simulink model "day4"  (R2024a)
settings: Solver=VariableStepAuto  StartTime=0.0  StopTime=10.0  RelTol=1e-3
libraries: simulink_extras x17
settings Model: Creator=tusha  LastModifiedBy=tusha

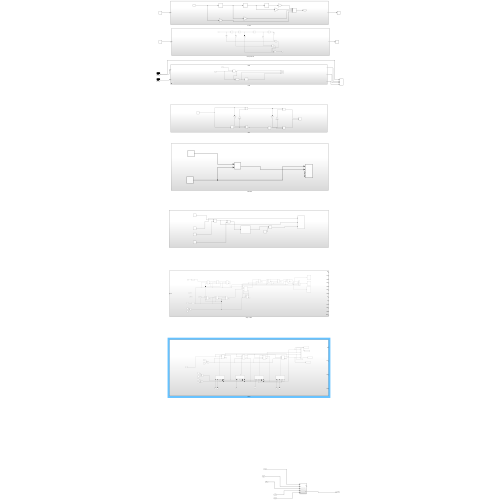
[thumbnail: Simulink's stored preview of the top-level diagram]
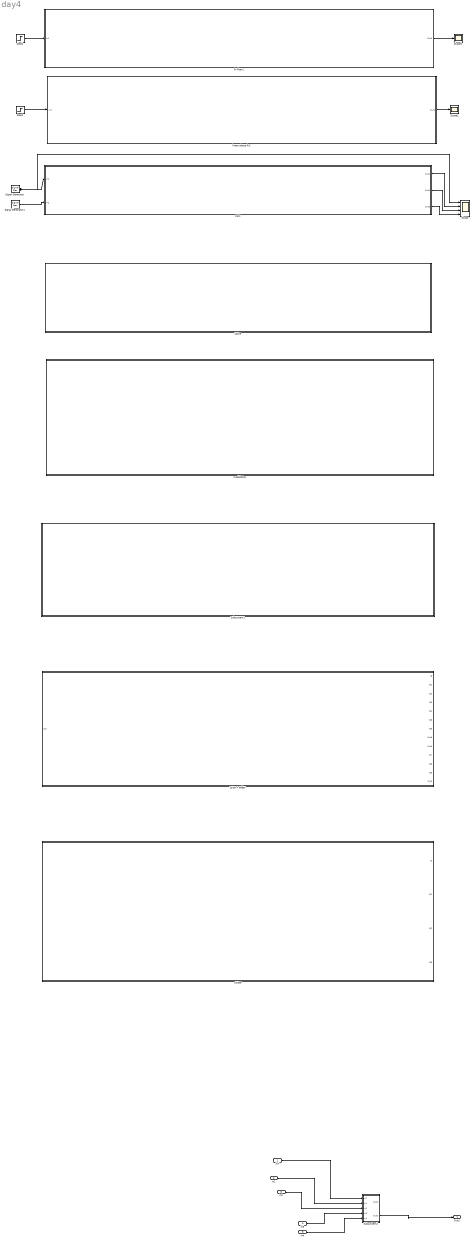
== system day4 ==
  In7 : Inport
  In1 : Inport  Port=2
  In2 : Inport  Port=3
  In3 : Inport  Port=4
  In4 : Inport  Port=5
  2sipo + adder : Subsystem
  PAM : Subsystem  Variant=on  VariantControlMode=label  VariantControl=PAM  LabelModeActiveChoice=PAM
  Scope : Scope  NumInputPorts=4
  Scope1 : Scope
  Scope2 : Scope
  Signal Generator : SignalGenerator  Units=rad/sec
  Signal Generator1 : SignalGenerator  WaveForm=square  Frequency=20  Units=rad/sec
  Step1 : Step  SampleTime=0
  Step2 : Step  SampleTime=0
  Subsystem1 : Subsystem
  Subsystem2 : Subsystem
  fir filter1 : Subsystem
  latice : Subsystem
  linear phase fir2 : Subsystem
  modulation : Subsystem
  shifter : Subsystem
  Out2 : Outport
  wires:
  Step1/1 -> fir filter1/1(In1)
  fir filter1/1(Out1) -> Scope1/1
  Step2/1 -> linear phase fir2/1(In1)
  linear phase fir2/1(Out1) -> Scope2/1
  Signal Generator/1 -> Scope/1, PAM/1(In1)
  Signal Generator1/1 -> PAM/2(In2)
  PAM/1(Out1) -> Scope/2
  PAM/2(Out2) -> Scope/3
  PAM/3(Out3) -> Scope/4
  In3/1 -> Subsystem2/4(In3)
  Subsystem2/2(Out2) -> Out2/1
  In1/1 -> Subsystem2/2(In1)
  In7/1 -> Subsystem2/1(In7)
  In2/1 -> Subsystem2/3(In2)
  In4/1 -> Subsystem2/5(In4)

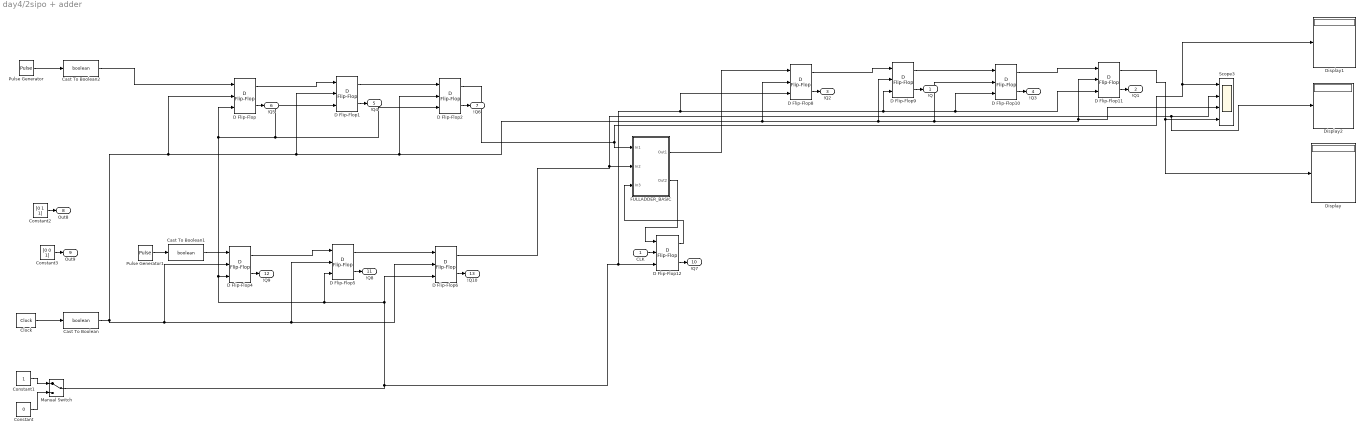
== system day4/2sipo + adder ==
  CLK : Inport
  Cast To Boolean : DataTypeConversion  OutDataTypeStr=boolean  SaturateOnIntegerOverflow=off  RndMeth=Floor
  Cast To Boolean1 : DataTypeConversion  OutDataTypeStr=boolean  SaturateOnIntegerOverflow=off  RndMeth=Floor
  Cast To Boolean2 : DataTypeConversion  OutDataTypeStr=boolean  SaturateOnIntegerOverflow=off  RndMeth=Floor
  Clock : simulink_extras/Flip Flops/Clock  period=0.5
  Constant : Constant  Value=0  OutDataTypeStr=boolean
  Constant1 : Constant  OutDataTypeStr=boolean
  Constant2 : Constant  Value=[0 1 1]
  Constant3 : Constant  Value=[0 0 1]
  D Flip-Flop{,1..2,4..6,8..12} (11 alike) : simulink_extras/Flip Flops/D Flip-Flop
  Display : Display
  Display1 : Display
  Display2 : Display
  FULLADDER_BASIC : Subsystem
  Manual Switch : ManualSwitch
  Pulse Generator : DiscretePulseGenerator  PulseType=Time based  PulseWidth=50
  Pulse Generator1 : DiscretePulseGenerator  PulseType=Time based  Period=1  PulseWidth=50
  Scope3 : Scope  NumInputPorts=4
  !Q : Outport
  !Q1 : Outport  Port=2
  !Q2 : Outport  Port=3
  !Q3 : Outport  Port=4
  !Q4 : Outport  Port=5
  !Q5 : Outport  Port=6
  !Q6 : Outport  Port=7
  Out8 : Outport  Port=8
  Out9 : Outport  Port=9
  !Q7 : Outport  Port=10
  !Q8 : Outport  Port=11
  !Q9 : Outport  Port=12
  !Q10 : Outport  Port=13
  wires:
  Cast To Boolean/1 -> D Flip-Flop6/2, D Flip-Flop5/2, D Flip-Flop4/2, Scope3/3, D Flip-Flop11/2, D Flip-Flop10/2, D Flip-Flop9/2, D Flip-Flop8/2, D Flip-Flop2/2, D Flip-Flop1/2, D Flip-Flop/2
  D Flip-Flop10/1 -> D Flip-Flop11/1
  Manual Switch/1 -> D Flip-Flop8/3, D Flip-Flop9/3, D Flip-Flop10/3, D Flip-Flop11/3, D Flip-Flop12/3, D Flip-Flop6/3, D Flip-Flop2/3, D Flip-Flop1/3, D Flip-Flop/3, D Flip-Flop4/3, D Flip-Flop5/3
  D Flip-Flop8/1 -> D Flip-Flop9/1
  D Flip-Flop11/1 -> Scope3/4, Display/1
  Pulse Generator/1 -> Cast To Boolean2/1
  Clock/1 -> Cast To Boolean/1
  D Flip-Flop4/1 -> D Flip-Flop5/1
  Constant2/1 -> Out8/1
  Cast To Boolean2/1 -> D Flip-Flop/1
  D Flip-Flop9/1 -> D Flip-Flop10/1
  D Flip-Flop5/1 -> D Flip-Flop6/1
  D Flip-Flop1/1 -> D Flip-Flop2/1
  D Flip-Flop6/1 -> FULLADDER_BASIC/2(In2), Scope3/2, Display2/1
  D Flip-Flop2/1 -> FULLADDER_BASIC/1(In1), Scope3/1, Display1/1
  D Flip-Flop/1 -> D Flip-Flop1/1
  Constant/1 -> Manual Switch/2
  D Flip-Flop8/2 -> !Q2/1
  D Flip-Flop12/1 -> FULLADDER_BASIC/3(In3)
  Pulse Generator1/1 -> Cast To Boolean1/1
  FULLADDER_BASIC/2(Out2) -> D Flip-Flop12/1
  FULLADDER_BASIC/1(Out1) -> D Flip-Flop8/1
  Constant1/1 -> Manual Switch/1
  Cast To Boolean1/1 -> D Flip-Flop4/1
  D Flip-Flop10/2 -> !Q3/1
  D Flip-Flop11/2 -> !Q1/1
  D Flip-Flop4/2 -> !Q9/1
  D Flip-Flop9/2 -> !Q/1
  D Flip-Flop5/2 -> !Q8/1
  D Flip-Flop1/2 -> !Q4/1
  CLK/1 -> D Flip-Flop12/2
  D Flip-Flop6/2 -> !Q10/1
  D Flip-Flop12/2 -> !Q7/1
  D Flip-Flop/2 -> !Q5/1
  D Flip-Flop2/2 -> !Q6/1
  Constant3/1 -> Out9/1

== system day4/PAM ==
  In1 : Inport
  In2 : Inport  Port=2
  PAM : Subsystem  VariantControl=PAM
  Out1 : Outport
  Out2 : Outport  Port=2
  Out3 : Outport  Port=3

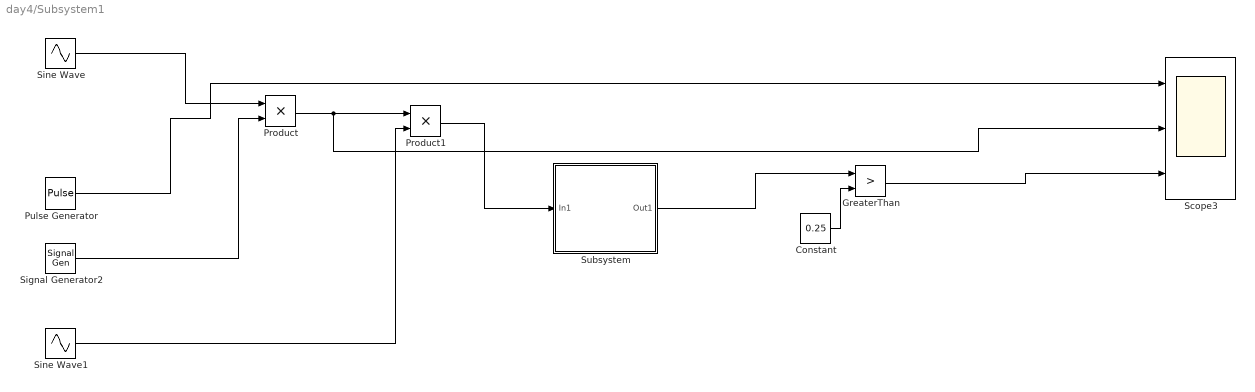
== system day4/Subsystem1 ==
  Constant : Constant  Value=0.25
  GreaterThan : RelationalOperator  Operator=>  OutDataTypeStr=boolean  RndMeth=Simplest  InputSameDT=off
  Product : Product
  Product1 : Product
  Pulse Generator : DiscretePulseGenerator  PulseType=Time based  Period=1  PulseWidth=50
  Scope3 : Scope  NumInputPorts=3
  Signal Generator2 : SignalGenerator  Units=rad/sec
  Sine Wave : Sin  Frequency=20  SampleTime=0
  Sine Wave1 : Sin  Frequency=20  SampleTime=0
  Subsystem : Subsystem
  wires:
  Pulse Generator/1 -> Scope3/1
  Sine Wave1/1 -> Product1/2
  Signal Generator2/1 -> Product/2
  Sine Wave/1 -> Product/1
  Subsystem/1(Out1) -> GreaterThan/1
  Product1/1 -> Subsystem/1(In1)
  Constant/1 -> GreaterThan/2
  Product/1 -> Scope3/2, Product1/1
  GreaterThan/1 -> Scope3/3

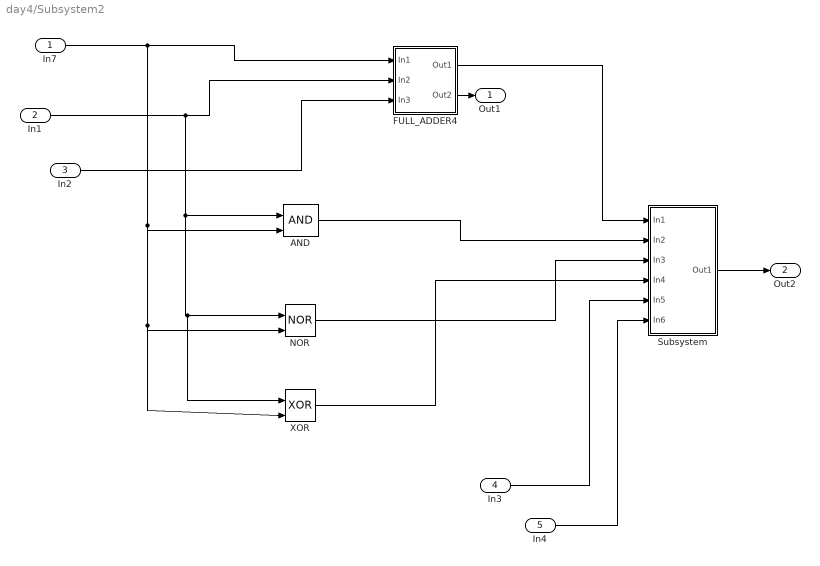
== system day4/Subsystem2 ==
  In7 : Inport
  In1 : Inport  Port=2
  In2 : Inport  Port=3
  In3 : Inport  Port=4
  In4 : Inport  Port=5
  AND : Logic  IconShape=distinctive  AllPortsSameDT=off  OutDataTypeStr=boolean
  FULL_ADDER4 : Subsystem
  NOR : Logic  Operator=NOR  IconShape=distinctive  AllPortsSameDT=off  OutDataTypeStr=boolean
  Subsystem : Subsystem
  XOR : Logic  Operator=XOR  IconShape=distinctive  AllPortsSameDT=off  OutDataTypeStr=boolean
  Out1 : Outport
  Out2 : Outport  Port=2
  wires:
  In7/1 -> XOR/2, NOR/2, AND/2, FULL_ADDER4/1(In1)
  Subsystem/1(Out1) -> Out2/1
  FULL_ADDER4/1(Out1) -> Subsystem/1(In1)
  In4/1 -> Subsystem/6(In6)
  In1/1 -> XOR/1, NOR/1, AND/1, FULL_ADDER4/2(In2)
  In2/1 -> FULL_ADDER4/3(In3)
  XOR/1 -> Subsystem/4(In4)
  AND/1 -> Subsystem/2(In2)
  NOR/1 -> Subsystem/3(In3)
  In3/1 -> Subsystem/5(In5)
  FULL_ADDER4/2(Out2) -> Out1/1

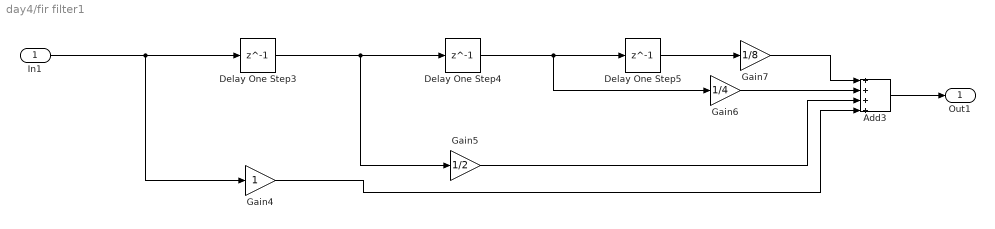
== system day4/fir filter1 ==
  In1 : Inport
  Add3 : Sum  Inputs=++++
  Delay One Step3 : Delay  DelayLength=1
  Delay One Step4 : Delay  DelayLength=1
  Delay One Step5 : Delay  DelayLength=1
  Gain4 : Gain
  Gain5 : Gain  Gain=1/2
  Gain6 : Gain  Gain=1/4
  Gain7 : Gain  Gain=1/8
  Out1 : Outport
  wires:
  Delay One Step5/1 -> Gain7/1
  Delay One Step4/1 -> Delay One Step5/1, Gain6/1
  Gain4/1 -> Add3/4
  Gain7/1 -> Add3/1
  Delay One Step3/1 -> Delay One Step4/1, Gain5/1
  Gain6/1 -> Add3/2
  Gain5/1 -> Add3/3
  In1/1 -> Gain4/1, Delay One Step3/1
  Add3/1 -> Out1/1

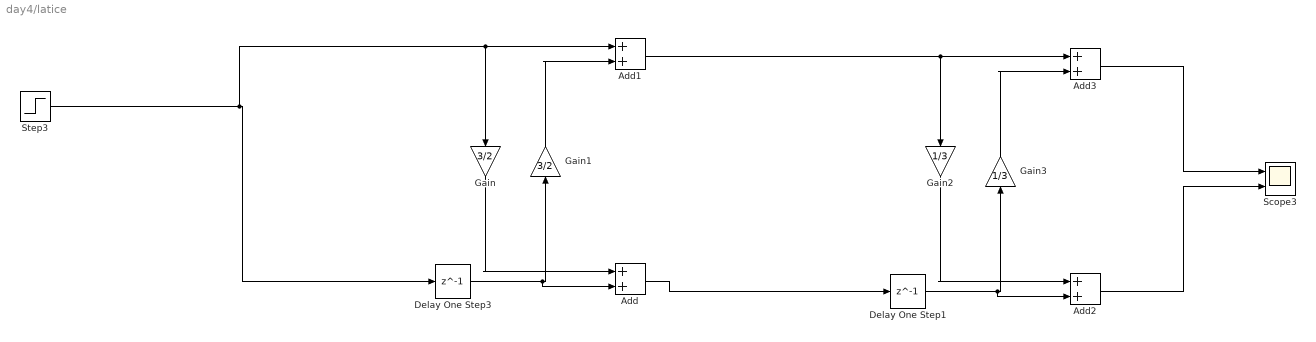
== system day4/latice ==
  Add{,1..3} (4 alike) : Sum
  Delay One Step1 : Delay  DelayLength=1
  Delay One Step3 : Delay  DelayLength=1
  Gain : Gain  Gain=3/2
  Gain1 : Gain  Gain=3/2
  Gain2 : Gain  Gain=1/3
  Gain3 : Gain  Gain=1/3
  Scope3 : Scope  NumInputPorts=2
  Step3 : Step  SampleTime=0
  wires:
  Add2/1 -> Scope3/2
  Gain1/1 -> Add1/2
  Gain3/1 -> Add3/2
  Step3/1 -> Gain/1, Add1/1, Delay One Step3/1
  Delay One Step3/1 -> Add/2, Gain1/1
  Gain/1 -> Add/1
  Add/1 -> Delay One Step1/1
  Delay One Step1/1 -> Add2/2, Gain3/1
  Add3/1 -> Scope3/1
  Gain2/1 -> Add2/1
  Add1/1 -> Gain2/1, Add3/1

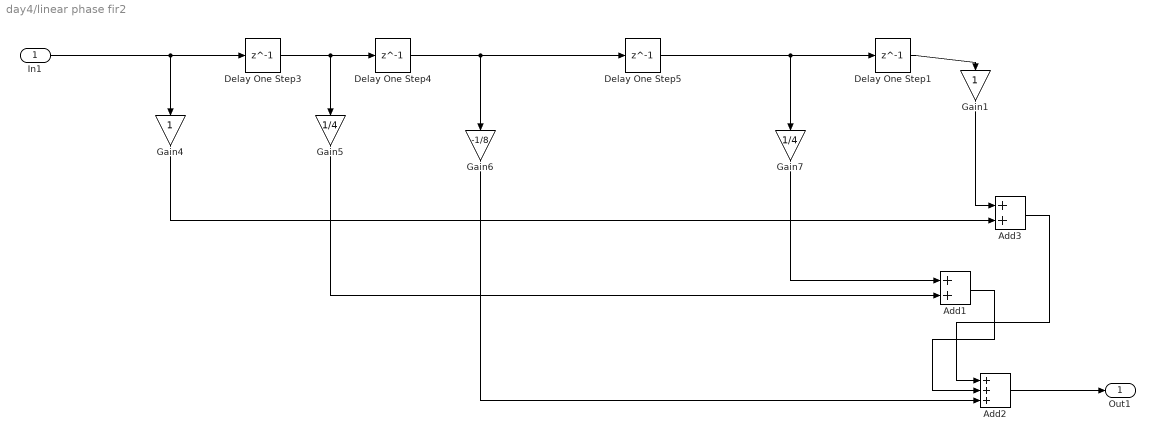
== system day4/linear phase fir2 ==
  In1 : Inport
  Add1 : Sum
  Add2 : Sum  Inputs=+++
  Add3 : Sum
  Delay One Step{1,3..5} (4 alike) : Delay  DelayLength=1
  Gain1 : Gain
  Gain4 : Gain
  Gain5 : Gain  Gain=1/4
  Gain6 : Gain  Gain=-1/8
  Gain7 : Gain  Gain=1/4
  Out1 : Outport
  wires:
  Delay One Step4/1 -> Delay One Step5/1, Gain6/1
  Add3/1 -> Add2/1
  Add1/1 -> Add2/2
  Delay One Step5/1 -> Delay One Step1/1, Gain7/1
  In1/1 -> Gain4/1, Delay One Step3/1
  Delay One Step3/1 -> Delay One Step4/1, Gain5/1
  Gain4/1 -> Add3/2
  Gain6/1 -> Add2/3
  Delay One Step1/1 -> Gain1/1
  Gain7/1 -> Add1/1
  Gain5/1 -> Add1/2
  Gain1/1 -> Add3/1
  Add2/1 -> Out1/1

== system day4/modulation ==
  Product : Product
  Pulse Generator : DiscretePulseGenerator  PulseType=Time based  Period=1  PulseWidth=50
  Scope3 : Scope  NumInputPorts=4
  Sine Wave : Sin  Frequency=50  SampleTime=0
  wires:
  Sine Wave/1 -> Product/1
  Pulse Generator/1 -> Scope3/1, Product/2
  Product/1 -> Scope3/2

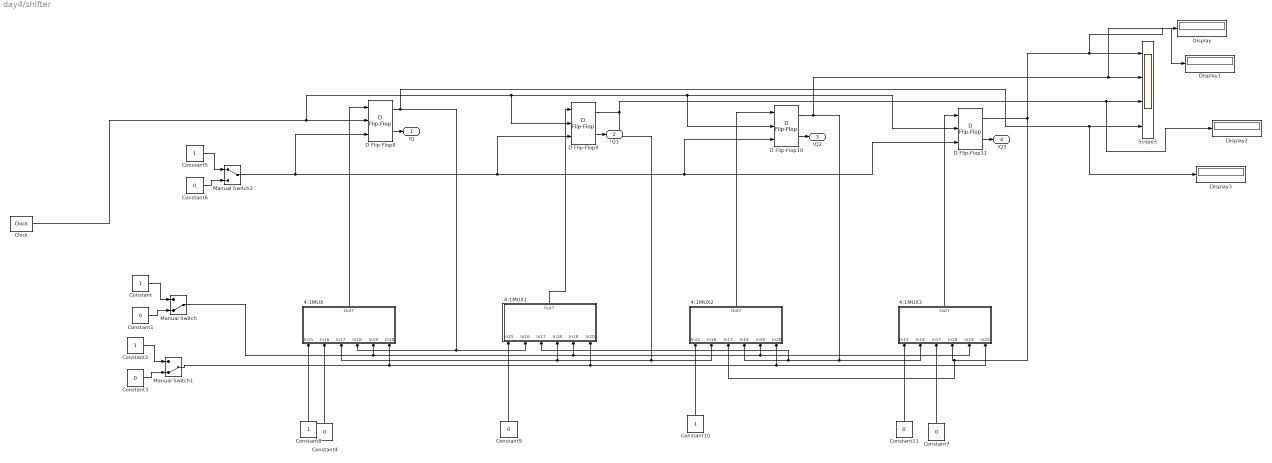
== system day4/shifter ==
  4:1MUX : Subsystem
  4:1MUX1 : Subsystem
  4:1MUX2 : Subsystem
  4:1MUX3 : Subsystem
  Clock : simulink_extras/Flip Flops/Clock  period=2
  Constant{,2,5,8,10} (5 alike) : Constant
  Constant{1,3..4,6..7,9,11} (7 alike) : Constant  Value=0
  D Flip-Flop{8..11} (4 alike) : simulink_extras/Flip Flops/D Flip-Flop
  Display{,1..3} (4 alike) : Display
  Manual Switch : ManualSwitch  CurrentSetting=0
  Manual Switch1 : ManualSwitch  CurrentSetting=0
  Manual Switch2 : ManualSwitch
  Scope3 : Scope  NumInputPorts=4
  !Q : Outport
  !Q1 : Outport  Port=2
  !Q2 : Outport  Port=3
  !Q3 : Outport  Port=4
  wires:
  4:1MUX2/1(Out7) -> D Flip-Flop10/1
  Constant/1 -> Manual Switch/1
  Constant8/1 -> 4:1MUX/1(In15)
  Manual Switch2/1 -> D Flip-Flop11/3, D Flip-Flop10/3, D Flip-Flop9/3, D Flip-Flop8/3
  Manual Switch/1 -> 4:1MUX3/5(In19), 4:1MUX2/5(In19), 4:1MUX1/5(In19), 4:1MUX/5(In19)
  4:1MUX3/1(Out7) -> D Flip-Flop11/1
  D Flip-Flop11/1 -> 4:1MUX2/3(In17), 4:1MUX3/4(In18), Display/1, Scope3/1
  D Flip-Flop9/1 -> 4:1MUX/3(In17), 4:1MUX1/4(In18), 4:1MUX2/2(In16), Display2/1, Scope3/3
  D Flip-Flop9/2 -> !Q1/1
  4:1MUX1/1(Out7) -> D Flip-Flop9/1
  Manual Switch1/1 -> 4:1MUX/6(In20), 4:1MUX1/6(In20), 4:1MUX3/6(In20), 4:1MUX2/6(In20)
  D Flip-Flop10/1 -> Display1/1, Scope3/2, 4:1MUX1/3(In17), 4:1MUX2/4(In18), 4:1MUX3/2(In16)
  Constant3/1 -> Manual Switch1/2
  D Flip-Flop8/1 -> Display3/1, Scope3/4, 4:1MUX1/2(In16), 4:1MUX/4(In18)
  Constant6/1 -> Manual Switch2/2
  Constant2/1 -> Manual Switch1/1
  Constant5/1 -> Manual Switch2/1
  Constant9/1 -> 4:1MUX1/1(In15)
  Clock/1 -> D Flip-Flop10/2, D Flip-Flop11/2, D Flip-Flop9/2, D Flip-Flop8/2
  Constant7/1 -> 4:1MUX3/3(In17)
  Constant4/1 -> 4:1MUX/2(In16)
  Constant1/1 -> Manual Switch/2
  4:1MUX/1(Out7) -> D Flip-Flop8/1
  Constant10/1 -> 4:1MUX2/1(In15)
  Constant11/1 -> 4:1MUX3/1(In15)
  D Flip-Flop10/2 -> !Q2/1
  D Flip-Flop11/2 -> !Q3/1
  D Flip-Flop8/2 -> !Q/1

== system day4/2sipo + adder/FULLADDER_BASIC ==
  In1 : Inport
  In2 : Inport  Port=2
  In3 : Inport  Port=3
  HA_Basic1 : Subsystem
  HA_Basic2 : Subsystem
  Logical Operator4 : Logic  Operator=OR  IconShape=distinctive  AllPortsSameDT=off  OutDataTypeStr=boolean
  Out1 : Outport
  Out2 : Outport  Port=2
  wires:
  HA_Basic1/1(Out1) -> HA_Basic2/1(In1)
  HA_Basic1/2(Out2) -> Logical Operator4/2
  HA_Basic2/2(Out2) -> Logical Operator4/1
  In1/1 -> HA_Basic1/1(In1)
  Logical Operator4/1 -> Out2/1
  In2/1 -> HA_Basic1/2(In2)
  HA_Basic2/1(Out1) -> Out1/1
  In3/1 -> HA_Basic2/2(In2)

== system day4/PAM/PAM ==
  In1 : Inport
  In2 : Inport  Port=2
  Product : Product
  Product1 : Product
  fir filter2 : Subsystem
  Out1 : Outport
  Out2 : Outport  Port=2
  Out3 : Outport  Port=3
  wires:
  fir filter2/1(Out1) -> Out3/1
  Product/1 -> Out1/1, Product1/1
  In2/1 -> Product/2, Product1/2
  In1/1 -> Product/1
  Product1/1 -> Out2/1, fir filter2/1(In1)

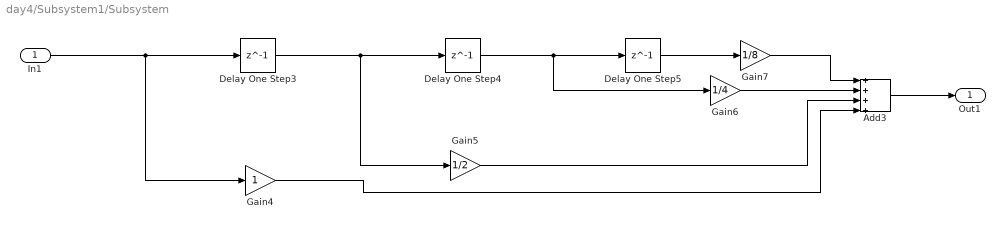
== system day4/Subsystem1/Subsystem ==
  In1 : Inport
  Add3 : Sum  Inputs=++++
  Delay One Step3 : Delay  DelayLength=1
  Delay One Step4 : Delay  DelayLength=1
  Delay One Step5 : Delay  DelayLength=1
  Gain4 : Gain
  Gain5 : Gain  Gain=1/2
  Gain6 : Gain  Gain=1/4
  Gain7 : Gain  Gain=1/8
  Out1 : Outport
  wires:
  Gain6/1 -> Add3/2
  In1/1 -> Gain4/1, Delay One Step3/1
  Delay One Step4/1 -> Delay One Step5/1, Gain6/1
  Gain4/1 -> Add3/4
  Gain5/1 -> Add3/3
  Delay One Step5/1 -> Gain7/1
  Delay One Step3/1 -> Delay One Step4/1, Gain5/1
  Gain7/1 -> Add3/1
  Add3/1 -> Out1/1

== system day4/Subsystem2/FULL_ADDER4 ==
  In1 : Inport
  In2 : Inport  Port=2
  In3 : Inport  Port=3
  Logical Operator : Logic  Operator=OR  AllPortsSameDT=off  OutDataTypeStr=boolean
  half_adder : Subsystem
  half_adder1 : Subsystem
  Out1 : Outport
  Out2 : Outport  Port=2
  wires:
  half_adder1/2(Out2) -> Logical Operator/2
  In3/1 -> half_adder1/2(In2)
  In1/1 -> half_adder/1(In1)
  half_adder1/1(Out1) -> Out1/1
  half_adder/1(Out1) -> half_adder1/1(In1)
  half_adder/2(Out2) -> Logical Operator/1
  In2/1 -> half_adder/2(In2)
  Logical Operator/1 -> Out2/1

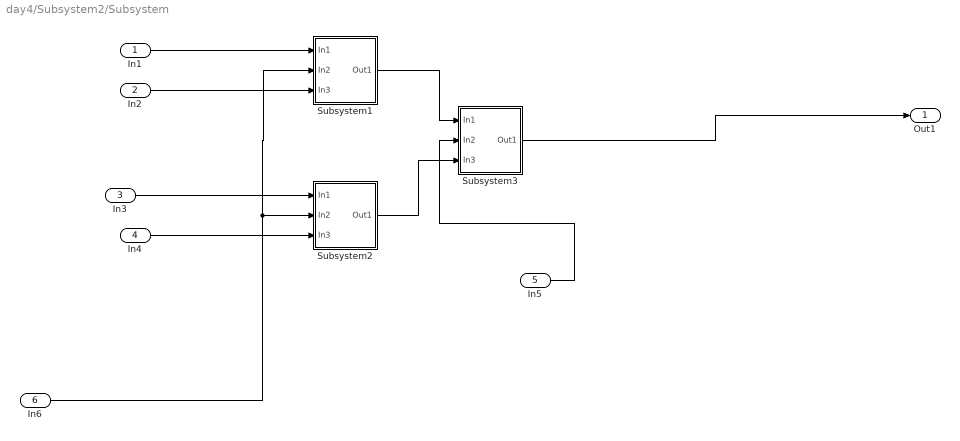
== system day4/Subsystem2/Subsystem ==
  In1 : Inport
  In2 : Inport  Port=2
  In3 : Inport  Port=3
  In4 : Inport  Port=4
  In5 : Inport  Port=5
  In6 : Inport  Port=6
  Subsystem1 : Subsystem
  Subsystem2 : Subsystem
  Subsystem3 : Subsystem
  Out1 : Outport
  wires:
  In6/1 -> Subsystem1/2(In2), Subsystem2/2(In2)
  In2/1 -> Subsystem1/3(In3)
  In3/1 -> Subsystem2/1(In1)
  Subsystem2/1(Out1) -> Subsystem3/3(In3)
  Subsystem1/1(Out1) -> Subsystem3/1(In1)
  In4/1 -> Subsystem2/3(In3)
  In1/1 -> Subsystem1/1(In1)
  In5/1 -> Subsystem3/2(In2)
  Subsystem3/1(Out1) -> Out1/1

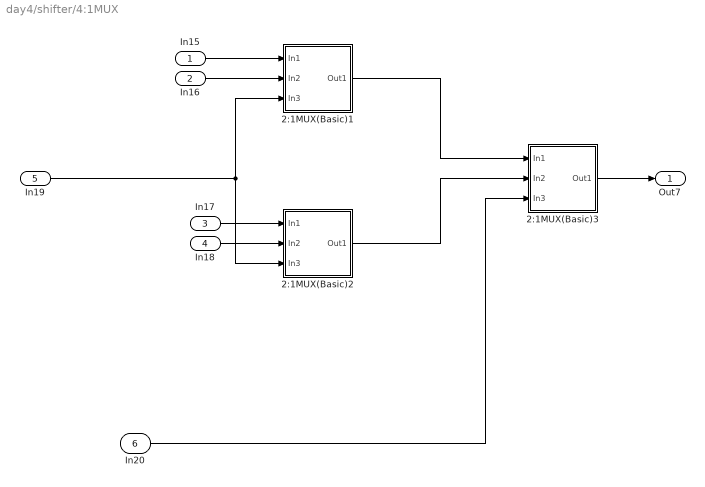
== system day4/shifter/4:1MUX ==
  In15 : Inport
  In16 : Inport  Port=2
  In17 : Inport  Port=3
  In18 : Inport  Port=4
  In19 : Inport  Port=5
  In20 : Inport  Port=6
  2:1MUX(Basic)1 : Subsystem
  2:1MUX(Basic)2 : Subsystem
  2:1MUX(Basic)3 : Subsystem
  Out7 : Outport
  wires:
  In18/1 -> 2:1MUX(Basic)2/2(In2)
  In16/1 -> 2:1MUX(Basic)1/2(In2)
  In17/1 -> 2:1MUX(Basic)2/1(In1)
  In19/1 -> 2:1MUX(Basic)2/3(In3), 2:1MUX(Basic)1/3(In3)
  2:1MUX(Basic)2/1(Out1) -> 2:1MUX(Basic)3/2(In2)
  2:1MUX(Basic)1/1(Out1) -> 2:1MUX(Basic)3/1(In1)
  In20/1 -> 2:1MUX(Basic)3/3(In3)
  In15/1 -> 2:1MUX(Basic)1/1(In1)
  2:1MUX(Basic)3/1(Out1) -> Out7/1

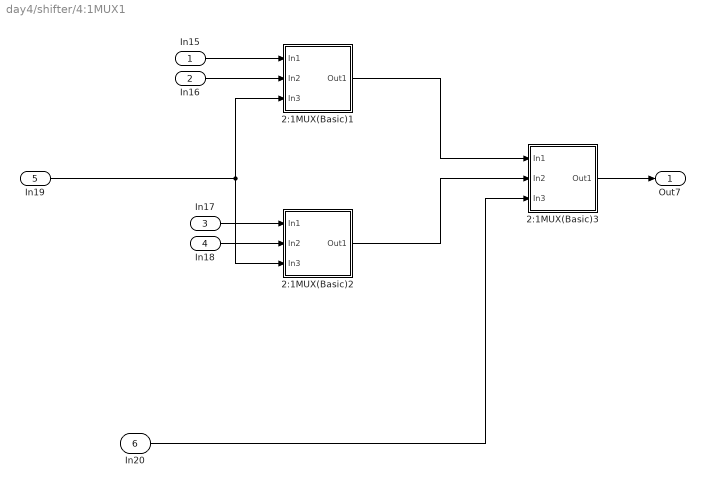
== system day4/shifter/4:1MUX1 ==
  In15 : Inport
  In16 : Inport  Port=2
  In17 : Inport  Port=3
  In18 : Inport  Port=4
  In19 : Inport  Port=5
  In20 : Inport  Port=6
  2:1MUX(Basic)1 : Subsystem
  2:1MUX(Basic)2 : Subsystem
  2:1MUX(Basic)3 : Subsystem
  Out7 : Outport
  wires:
  In18/1 -> 2:1MUX(Basic)2/2(In2)
  In16/1 -> 2:1MUX(Basic)1/2(In2)
  In17/1 -> 2:1MUX(Basic)2/1(In1)
  In19/1 -> 2:1MUX(Basic)2/3(In3), 2:1MUX(Basic)1/3(In3)
  2:1MUX(Basic)2/1(Out1) -> 2:1MUX(Basic)3/2(In2)
  2:1MUX(Basic)1/1(Out1) -> 2:1MUX(Basic)3/1(In1)
  In20/1 -> 2:1MUX(Basic)3/3(In3)
  In15/1 -> 2:1MUX(Basic)1/1(In1)
  2:1MUX(Basic)3/1(Out1) -> Out7/1

== system day4/shifter/4:1MUX2 ==
  In15 : Inport
  In16 : Inport  Port=2
  In17 : Inport  Port=3
  In18 : Inport  Port=4
  In19 : Inport  Port=5
  In20 : Inport  Port=6
  2:1MUX(Basic)1 : Subsystem
  2:1MUX(Basic)2 : Subsystem
  2:1MUX(Basic)3 : Subsystem
  Out7 : Outport
  wires:
  In18/1 -> 2:1MUX(Basic)2/2(In2)
  In16/1 -> 2:1MUX(Basic)1/2(In2)
  In17/1 -> 2:1MUX(Basic)2/1(In1)
  In19/1 -> 2:1MUX(Basic)2/3(In3), 2:1MUX(Basic)1/3(In3)
  2:1MUX(Basic)2/1(Out1) -> 2:1MUX(Basic)3/2(In2)
  2:1MUX(Basic)1/1(Out1) -> 2:1MUX(Basic)3/1(In1)
  In20/1 -> 2:1MUX(Basic)3/3(In3)
  In15/1 -> 2:1MUX(Basic)1/1(In1)
  2:1MUX(Basic)3/1(Out1) -> Out7/1

== system day4/shifter/4:1MUX3 ==
  In15 : Inport
  In16 : Inport  Port=2
  In17 : Inport  Port=3
  In18 : Inport  Port=4
  In19 : Inport  Port=5
  In20 : Inport  Port=6
  2:1MUX(Basic)1 : Subsystem
  2:1MUX(Basic)2 : Subsystem
  2:1MUX(Basic)3 : Subsystem
  Out7 : Outport
  wires:
  In18/1 -> 2:1MUX(Basic)2/2(In2)
  In16/1 -> 2:1MUX(Basic)1/2(In2)
  In17/1 -> 2:1MUX(Basic)2/1(In1)
  In19/1 -> 2:1MUX(Basic)2/3(In3), 2:1MUX(Basic)1/3(In3)
  2:1MUX(Basic)2/1(Out1) -> 2:1MUX(Basic)3/2(In2)
  2:1MUX(Basic)1/1(Out1) -> 2:1MUX(Basic)3/1(In1)
  In20/1 -> 2:1MUX(Basic)3/3(In3)
  In15/1 -> 2:1MUX(Basic)1/1(In1)
  2:1MUX(Basic)3/1(Out1) -> Out7/1

== system day4/2sipo + adder/FULLADDER_BASIC/HA_Basic1 ==
  In1 : Inport
  In2 : Inport  Port=2
  Logical Operator2 : Logic  IconShape=distinctive  AllPortsSameDT=off  OutDataTypeStr=boolean
  XOR_basic1 : Subsystem
  Out1 : Outport
  Out2 : Outport  Port=2
  wires:
  XOR_basic1/1(Out1) -> Out1/1
  Logical Operator2/1 -> Out2/1
  In1/1 -> Logical Operator2/1, XOR_basic1/1(In1)
  In2/1 -> Logical Operator2/2, XOR_basic1/2(In2)

== system day4/2sipo + adder/FULLADDER_BASIC/HA_Basic2 ==
  In1 : Inport
  In2 : Inport  Port=2
  Logical Operator2 : Logic  IconShape=distinctive  AllPortsSameDT=off  OutDataTypeStr=boolean
  XOR_basic1 : Subsystem
  Out1 : Outport
  Out2 : Outport  Port=2
  wires:
  XOR_basic1/1(Out1) -> Out1/1
  Logical Operator2/1 -> Out2/1
  In1/1 -> Logical Operator2/1, XOR_basic1/1(In1)
  In2/1 -> Logical Operator2/2, XOR_basic1/2(In2)

== system day4/PAM/PAM/fir filter2 ==
  In1 : Inport
  Add3 : Sum  Inputs=++++
  Delay One Step3 : Delay  DelayLength=1
  Delay One Step4 : Delay  DelayLength=1
  Delay One Step5 : Delay  DelayLength=1
  Gain4 : Gain
  Gain5 : Gain  Gain=1/2
  Gain6 : Gain  Gain=1/4
  Gain7 : Gain  Gain=1/8
  Out1 : Outport
  wires:
  Delay One Step5/1 -> Gain7/1
  Delay One Step4/1 -> Delay One Step5/1, Gain6/1
  Gain4/1 -> Add3/4
  Gain7/1 -> Add3/1
  Delay One Step3/1 -> Delay One Step4/1, Gain5/1
  Gain6/1 -> Add3/2
  Gain5/1 -> Add3/3
  In1/1 -> Gain4/1, Delay One Step3/1
  Add3/1 -> Out1/1

== system day4/Subsystem2/FULL_ADDER4/half_adder ==
  In1 : Inport
  In2 : Inport  Port=2
  Logical Operator1 : Logic  AllPortsSameDT=off  OutDataTypeStr=boolean
  XOR_BASIC : Subsystem
  Out1 : Outport
  Out2 : Outport  Port=2
  wires:
  In1/1 -> XOR_BASIC/1(In1), Logical Operator1/1
  In2/1 -> XOR_BASIC/2(In2), Logical Operator1/2
  Logical Operator1/1 -> Out2/1
  XOR_BASIC/1(Out1) -> Out1/1

== system day4/Subsystem2/FULL_ADDER4/half_adder1 ==
  In1 : Inport
  In2 : Inport  Port=2
  Logical Operator1 : Logic  AllPortsSameDT=off  OutDataTypeStr=boolean
  XOR_BASIC : Subsystem
  Out1 : Outport
  Out2 : Outport  Port=2
  wires:
  In1/1 -> XOR_BASIC/1(In1), Logical Operator1/1
  In2/1 -> XOR_BASIC/2(In2), Logical Operator1/2
  Logical Operator1/1 -> Out2/1
  XOR_BASIC/1(Out1) -> Out1/1

== system day4/Subsystem2/Subsystem/Subsystem1 ==
  In1 : Inport
  In2 : Inport  Port=2
  In3 : Inport  Port=3
  Logical Operator{,1..3} (4 alike) : Logic  Operator=NAND  AllPortsSameDT=off  OutDataTypeStr=boolean
  Out1 : Outport
  wires:
  Logical Operator2/1 -> Out1/1
  Logical Operator/1 -> Logical Operator1/1
  In2/1 -> Logical Operator/2, Logical Operator/1, Logical Operator3/2
  Logical Operator1/1 -> Logical Operator2/1
  In1/1 -> Logical Operator1/2
  Logical Operator3/1 -> Logical Operator2/2
  In3/1 -> Logical Operator3/1

== system day4/Subsystem2/Subsystem/Subsystem2 ==
  In1 : Inport
  In2 : Inport  Port=2
  In3 : Inport  Port=3
  Logical Operator{,1..3} (4 alike) : Logic  Operator=NAND  AllPortsSameDT=off  OutDataTypeStr=boolean
  Out1 : Outport
  wires:
  Logical Operator2/1 -> Out1/1
  Logical Operator/1 -> Logical Operator1/1
  In2/1 -> Logical Operator/2, Logical Operator/1, Logical Operator3/2
  Logical Operator1/1 -> Logical Operator2/1
  In1/1 -> Logical Operator1/2
  Logical Operator3/1 -> Logical Operator2/2
  In3/1 -> Logical Operator3/1

== system day4/Subsystem2/Subsystem/Subsystem3 ==
  In1 : Inport
  In2 : Inport  Port=2
  In3 : Inport  Port=3
  Logical Operator{,1..3} (4 alike) : Logic  Operator=NAND  AllPortsSameDT=off  OutDataTypeStr=boolean
  Out1 : Outport
  wires:
  Logical Operator2/1 -> Out1/1
  Logical Operator/1 -> Logical Operator1/1
  In2/1 -> Logical Operator/2, Logical Operator/1, Logical Operator3/2
  Logical Operator1/1 -> Logical Operator2/1
  In1/1 -> Logical Operator1/2
  Logical Operator3/1 -> Logical Operator2/2
  In3/1 -> Logical Operator3/1

== system day4/shifter/4:1MUX/2:1MUX(Basic)1 ==
  In1 : Inport
  In2 : Inport  Port=2
  In3 : Inport  Port=3
  Logical Operator10 : Logic  IconShape=distinctive  AllPortsSameDT=off  OutDataTypeStr=boolean
  Logical Operator11 : Logic  Operator=NOT  IconShape=distinctive  AllPortsSameDT=off  OutDataTypeStr=boolean
  Logical Operator8 : Logic  IconShape=distinctive  AllPortsSameDT=off  OutDataTypeStr=boolean
  Logical Operator9 : Logic  Operator=OR  IconShape=distinctive  AllPortsSameDT=off  OutDataTypeStr=boolean
  Out1 : Outport
  wires:
  In2/1 -> Logical Operator10/1
  Logical Operator8/1 -> Logical Operator9/1
  Logical Operator9/1 -> Out1/1
  In1/1 -> Logical Operator8/1
  Logical Operator10/1 -> Logical Operator9/2
  Logical Operator11/1 -> Logical Operator8/2
  In3/1 -> Logical Operator10/2, Logical Operator11/1

== system day4/shifter/4:1MUX/2:1MUX(Basic)2 ==
  In1 : Inport
  In2 : Inport  Port=2
  In3 : Inport  Port=3
  Logical Operator10 : Logic  IconShape=distinctive  AllPortsSameDT=off  OutDataTypeStr=boolean
  Logical Operator11 : Logic  Operator=NOT  IconShape=distinctive  AllPortsSameDT=off  OutDataTypeStr=boolean
  Logical Operator8 : Logic  IconShape=distinctive  AllPortsSameDT=off  OutDataTypeStr=boolean
  Logical Operator9 : Logic  Operator=OR  IconShape=distinctive  AllPortsSameDT=off  OutDataTypeStr=boolean
  Out1 : Outport
  wires:
  In2/1 -> Logical Operator10/1
  Logical Operator8/1 -> Logical Operator9/1
  Logical Operator9/1 -> Out1/1
  In1/1 -> Logical Operator8/1
  Logical Operator10/1 -> Logical Operator9/2
  Logical Operator11/1 -> Logical Operator8/2
  In3/1 -> Logical Operator10/2, Logical Operator11/1

== system day4/shifter/4:1MUX/2:1MUX(Basic)3 ==
  In1 : Inport
  In2 : Inport  Port=2
  In3 : Inport  Port=3
  Logical Operator10 : Logic  IconShape=distinctive  AllPortsSameDT=off  OutDataTypeStr=boolean
  Logical Operator11 : Logic  Operator=NOT  IconShape=distinctive  AllPortsSameDT=off  OutDataTypeStr=boolean
  Logical Operator8 : Logic  IconShape=distinctive  AllPortsSameDT=off  OutDataTypeStr=boolean
  Logical Operator9 : Logic  Operator=OR  IconShape=distinctive  AllPortsSameDT=off  OutDataTypeStr=boolean
  Out1 : Outport
  wires:
  In2/1 -> Logical Operator10/1
  Logical Operator8/1 -> Logical Operator9/1
  Logical Operator9/1 -> Out1/1
  In1/1 -> Logical Operator8/1
  Logical Operator10/1 -> Logical Operator9/2
  Logical Operator11/1 -> Logical Operator8/2
  In3/1 -> Logical Operator10/2, Logical Operator11/1

== system day4/shifter/4:1MUX1/2:1MUX(Basic)1 ==
  In1 : Inport
  In2 : Inport  Port=2
  In3 : Inport  Port=3
  Logical Operator10 : Logic  IconShape=distinctive  AllPortsSameDT=off  OutDataTypeStr=boolean
  Logical Operator11 : Logic  Operator=NOT  IconShape=distinctive  AllPortsSameDT=off  OutDataTypeStr=boolean
  Logical Operator8 : Logic  IconShape=distinctive  AllPortsSameDT=off  OutDataTypeStr=boolean
  Logical Operator9 : Logic  Operator=OR  IconShape=distinctive  AllPortsSameDT=off  OutDataTypeStr=boolean
  Out1 : Outport
  wires:
  In2/1 -> Logical Operator10/1
  Logical Operator8/1 -> Logical Operator9/1
  Logical Operator9/1 -> Out1/1
  In1/1 -> Logical Operator8/1
  Logical Operator10/1 -> Logical Operator9/2
  Logical Operator11/1 -> Logical Operator8/2
  In3/1 -> Logical Operator10/2, Logical Operator11/1

== system day4/shifter/4:1MUX1/2:1MUX(Basic)2 ==
  In1 : Inport
  In2 : Inport  Port=2
  In3 : Inport  Port=3
  Logical Operator10 : Logic  IconShape=distinctive  AllPortsSameDT=off  OutDataTypeStr=boolean
  Logical Operator11 : Logic  Operator=NOT  IconShape=distinctive  AllPortsSameDT=off  OutDataTypeStr=boolean
  Logical Operator8 : Logic  IconShape=distinctive  AllPortsSameDT=off  OutDataTypeStr=boolean
  Logical Operator9 : Logic  Operator=OR  IconShape=distinctive  AllPortsSameDT=off  OutDataTypeStr=boolean
  Out1 : Outport
  wires:
  In2/1 -> Logical Operator10/1
  Logical Operator8/1 -> Logical Operator9/1
  Logical Operator9/1 -> Out1/1
  In1/1 -> Logical Operator8/1
  Logical Operator10/1 -> Logical Operator9/2
  Logical Operator11/1 -> Logical Operator8/2
  In3/1 -> Logical Operator10/2, Logical Operator11/1

== system day4/shifter/4:1MUX1/2:1MUX(Basic)3 ==
  In1 : Inport
  In2 : Inport  Port=2
  In3 : Inport  Port=3
  Logical Operator10 : Logic  IconShape=distinctive  AllPortsSameDT=off  OutDataTypeStr=boolean
  Logical Operator11 : Logic  Operator=NOT  IconShape=distinctive  AllPortsSameDT=off  OutDataTypeStr=boolean
  Logical Operator8 : Logic  IconShape=distinctive  AllPortsSameDT=off  OutDataTypeStr=boolean
  Logical Operator9 : Logic  Operator=OR  IconShape=distinctive  AllPortsSameDT=off  OutDataTypeStr=boolean
  Out1 : Outport
  wires:
  In2/1 -> Logical Operator10/1
  Logical Operator8/1 -> Logical Operator9/1
  Logical Operator9/1 -> Out1/1
  In1/1 -> Logical Operator8/1
  Logical Operator10/1 -> Logical Operator9/2
  Logical Operator11/1 -> Logical Operator8/2
  In3/1 -> Logical Operator10/2, Logical Operator11/1

== system day4/shifter/4:1MUX2/2:1MUX(Basic)1 ==
  In1 : Inport
  In2 : Inport  Port=2
  In3 : Inport  Port=3
  Logical Operator10 : Logic  IconShape=distinctive  AllPortsSameDT=off  OutDataTypeStr=boolean
  Logical Operator11 : Logic  Operator=NOT  IconShape=distinctive  AllPortsSameDT=off  OutDataTypeStr=boolean
  Logical Operator8 : Logic  IconShape=distinctive  AllPortsSameDT=off  OutDataTypeStr=boolean
  Logical Operator9 : Logic  Operator=OR  IconShape=distinctive  AllPortsSameDT=off  OutDataTypeStr=boolean
  Out1 : Outport
  wires:
  In2/1 -> Logical Operator10/1
  Logical Operator8/1 -> Logical Operator9/1
  Logical Operator9/1 -> Out1/1
  In1/1 -> Logical Operator8/1
  Logical Operator10/1 -> Logical Operator9/2
  Logical Operator11/1 -> Logical Operator8/2
  In3/1 -> Logical Operator10/2, Logical Operator11/1

== system day4/shifter/4:1MUX2/2:1MUX(Basic)2 ==
  In1 : Inport
  In2 : Inport  Port=2
  In3 : Inport  Port=3
  Logical Operator10 : Logic  IconShape=distinctive  AllPortsSameDT=off  OutDataTypeStr=boolean
  Logical Operator11 : Logic  Operator=NOT  IconShape=distinctive  AllPortsSameDT=off  OutDataTypeStr=boolean
  Logical Operator8 : Logic  IconShape=distinctive  AllPortsSameDT=off  OutDataTypeStr=boolean
  Logical Operator9 : Logic  Operator=OR  IconShape=distinctive  AllPortsSameDT=off  OutDataTypeStr=boolean
  Out1 : Outport
  wires:
  In2/1 -> Logical Operator10/1
  Logical Operator8/1 -> Logical Operator9/1
  Logical Operator9/1 -> Out1/1
  In1/1 -> Logical Operator8/1
  Logical Operator10/1 -> Logical Operator9/2
  Logical Operator11/1 -> Logical Operator8/2
  In3/1 -> Logical Operator10/2, Logical Operator11/1

== system day4/shifter/4:1MUX2/2:1MUX(Basic)3 ==
  In1 : Inport
  In2 : Inport  Port=2
  In3 : Inport  Port=3
  Logical Operator10 : Logic  IconShape=distinctive  AllPortsSameDT=off  OutDataTypeStr=boolean
  Logical Operator11 : Logic  Operator=NOT  IconShape=distinctive  AllPortsSameDT=off  OutDataTypeStr=boolean
  Logical Operator8 : Logic  IconShape=distinctive  AllPortsSameDT=off  OutDataTypeStr=boolean
  Logical Operator9 : Logic  Operator=OR  IconShape=distinctive  AllPortsSameDT=off  OutDataTypeStr=boolean
  Out1 : Outport
  wires:
  In2/1 -> Logical Operator10/1
  Logical Operator8/1 -> Logical Operator9/1
  Logical Operator9/1 -> Out1/1
  In1/1 -> Logical Operator8/1
  Logical Operator10/1 -> Logical Operator9/2
  Logical Operator11/1 -> Logical Operator8/2
  In3/1 -> Logical Operator10/2, Logical Operator11/1

== system day4/shifter/4:1MUX3/2:1MUX(Basic)1 ==
  In1 : Inport
  In2 : Inport  Port=2
  In3 : Inport  Port=3
  Logical Operator10 : Logic  IconShape=distinctive  AllPortsSameDT=off  OutDataTypeStr=boolean
  Logical Operator11 : Logic  Operator=NOT  IconShape=distinctive  AllPortsSameDT=off  OutDataTypeStr=boolean
  Logical Operator8 : Logic  IconShape=distinctive  AllPortsSameDT=off  OutDataTypeStr=boolean
  Logical Operator9 : Logic  Operator=OR  IconShape=distinctive  AllPortsSameDT=off  OutDataTypeStr=boolean
  Out1 : Outport
  wires:
  In2/1 -> Logical Operator10/1
  Logical Operator8/1 -> Logical Operator9/1
  Logical Operator9/1 -> Out1/1
  In1/1 -> Logical Operator8/1
  Logical Operator10/1 -> Logical Operator9/2
  Logical Operator11/1 -> Logical Operator8/2
  In3/1 -> Logical Operator10/2, Logical Operator11/1

== system day4/shifter/4:1MUX3/2:1MUX(Basic)2 ==
  In1 : Inport
  In2 : Inport  Port=2
  In3 : Inport  Port=3
  Logical Operator10 : Logic  IconShape=distinctive  AllPortsSameDT=off  OutDataTypeStr=boolean
  Logical Operator11 : Logic  Operator=NOT  IconShape=distinctive  AllPortsSameDT=off  OutDataTypeStr=boolean
  Logical Operator8 : Logic  IconShape=distinctive  AllPortsSameDT=off  OutDataTypeStr=boolean
  Logical Operator9 : Logic  Operator=OR  IconShape=distinctive  AllPortsSameDT=off  OutDataTypeStr=boolean
  Out1 : Outport
  wires:
  In2/1 -> Logical Operator10/1
  Logical Operator8/1 -> Logical Operator9/1
  Logical Operator9/1 -> Out1/1
  In1/1 -> Logical Operator8/1
  Logical Operator10/1 -> Logical Operator9/2
  Logical Operator11/1 -> Logical Operator8/2
  In3/1 -> Logical Operator10/2, Logical Operator11/1

== system day4/shifter/4:1MUX3/2:1MUX(Basic)3 ==
  In1 : Inport
  In2 : Inport  Port=2
  In3 : Inport  Port=3
  Logical Operator10 : Logic  IconShape=distinctive  AllPortsSameDT=off  OutDataTypeStr=boolean
  Logical Operator11 : Logic  Operator=NOT  IconShape=distinctive  AllPortsSameDT=off  OutDataTypeStr=boolean
  Logical Operator8 : Logic  IconShape=distinctive  AllPortsSameDT=off  OutDataTypeStr=boolean
  Logical Operator9 : Logic  Operator=OR  IconShape=distinctive  AllPortsSameDT=off  OutDataTypeStr=boolean
  Out1 : Outport
  wires:
  In2/1 -> Logical Operator10/1
  Logical Operator8/1 -> Logical Operator9/1
  Logical Operator9/1 -> Out1/1
  In1/1 -> Logical Operator8/1
  Logical Operator10/1 -> Logical Operator9/2
  Logical Operator11/1 -> Logical Operator8/2
  In3/1 -> Logical Operator10/2, Logical Operator11/1

== system day4/2sipo + adder/FULLADDER_BASIC/HA_Basic1/XOR_basic1 ==
  In1 : Inport
  In2 : Inport  Port=2
  Logical Operator1 : Logic  IconShape=distinctive  AllPortsSameDT=off  OutDataTypeStr=boolean
  Logical Operator2 : Logic  IconShape=distinctive  AllPortsSameDT=off  OutDataTypeStr=boolean
  Logical Operator3 : Logic  Operator=NOT  IconShape=distinctive  AllPortsSameDT=off  OutDataTypeStr=boolean
  Logical Operator4 : Logic  Operator=OR  IconShape=distinctive  AllPortsSameDT=off  OutDataTypeStr=boolean
  Logical Operator5 : Logic  Operator=NOT  IconShape=distinctive  AllPortsSameDT=off  OutDataTypeStr=boolean
  Out1 : Outport
  wires:
  Logical Operator2/1 -> Logical Operator4/1
  Logical Operator3/1 -> Logical Operator2/1
  Logical Operator1/1 -> Logical Operator4/2
  In1/1 -> Logical Operator3/1, Logical Operator1/1
  Logical Operator4/1 -> Out1/1
  Logical Operator5/1 -> Logical Operator1/2
  In2/1 -> Logical Operator2/2, Logical Operator5/1

== system day4/2sipo + adder/FULLADDER_BASIC/HA_Basic2/XOR_basic1 ==
  In1 : Inport
  In2 : Inport  Port=2
  Logical Operator1 : Logic  IconShape=distinctive  AllPortsSameDT=off  OutDataTypeStr=boolean
  Logical Operator2 : Logic  IconShape=distinctive  AllPortsSameDT=off  OutDataTypeStr=boolean
  Logical Operator3 : Logic  Operator=NOT  IconShape=distinctive  AllPortsSameDT=off  OutDataTypeStr=boolean
  Logical Operator4 : Logic  Operator=OR  IconShape=distinctive  AllPortsSameDT=off  OutDataTypeStr=boolean
  Logical Operator5 : Logic  Operator=NOT  IconShape=distinctive  AllPortsSameDT=off  OutDataTypeStr=boolean
  Out1 : Outport
  wires:
  Logical Operator2/1 -> Logical Operator4/1
  Logical Operator3/1 -> Logical Operator2/1
  Logical Operator1/1 -> Logical Operator4/2
  In1/1 -> Logical Operator3/1, Logical Operator1/1
  Logical Operator4/1 -> Out1/1
  Logical Operator5/1 -> Logical Operator1/2
  In2/1 -> Logical Operator2/2, Logical Operator5/1

== system day4/Subsystem2/FULL_ADDER4/half_adder/XOR_BASIC ==
  In1 : Inport
  In2 : Inport  Port=2
  Logical Operator10 : Logic  Operator=NOT  IconShape=distinctive  AllPortsSameDT=off  OutDataTypeStr=boolean
  Logical Operator11 : Logic  Operator=NOT  IconShape=distinctive  AllPortsSameDT=off  OutDataTypeStr=boolean
  Logical Operator7 : Logic  IconShape=distinctive  AllPortsSameDT=off  OutDataTypeStr=boolean
  Logical Operator8 : Logic  IconShape=distinctive  AllPortsSameDT=off  OutDataTypeStr=boolean
  Logical Operator9 : Logic  Operator=OR  IconShape=distinctive  AllPortsSameDT=off  OutDataTypeStr=boolean
  Out1 : Outport
  wires:
  Logical Operator8/1 -> Logical Operator9/2
  Logical Operator7/1 -> Logical Operator9/1
  In2/1 -> Logical Operator7/2, Logical Operator11/1
  Logical Operator11/1 -> Logical Operator8/1
  Logical Operator9/1 -> Out1/1
  In1/1 -> Logical Operator8/2, Logical Operator10/1
  Logical Operator10/1 -> Logical Operator7/1

== system day4/Subsystem2/FULL_ADDER4/half_adder1/XOR_BASIC ==
  In1 : Inport
  In2 : Inport  Port=2
  Logical Operator10 : Logic  Operator=NOT  IconShape=distinctive  AllPortsSameDT=off  OutDataTypeStr=boolean
  Logical Operator11 : Logic  Operator=NOT  IconShape=distinctive  AllPortsSameDT=off  OutDataTypeStr=boolean
  Logical Operator7 : Logic  IconShape=distinctive  AllPortsSameDT=off  OutDataTypeStr=boolean
  Logical Operator8 : Logic  IconShape=distinctive  AllPortsSameDT=off  OutDataTypeStr=boolean
  Logical Operator9 : Logic  Operator=OR  IconShape=distinctive  AllPortsSameDT=off  OutDataTypeStr=boolean
  Out1 : Outport
  wires:
  Logical Operator8/1 -> Logical Operator9/2
  Logical Operator7/1 -> Logical Operator9/1
  In2/1 -> Logical Operator7/2, Logical Operator11/1
  Logical Operator11/1 -> Logical Operator8/1
  Logical Operator9/1 -> Out1/1
  In1/1 -> Logical Operator8/2, Logical Operator10/1
  Logical Operator10/1 -> Logical Operator7/1
